simulink model "AdaptiveQ_Function"  (R2025b)
settings: Solver=ode1  StartTime=0.0  StopTime=inf  FixedStep=0.002  RelTol=1e-3  EnableMultiTasking=on
undefined symbols (not defined in the file): A, B, P_ss_vec, Q, R
settings Model: SimulationMode=external  ExtModeTrigDuration=5000  Creator=MLevis  LastModifiedBy=mj
settings SolverCC: AlgebraicLoopSolver=TrustRegion  PositivePriorityOrder=on
settings DataIOCC: LimitDataPoints=on  SaveFormat=Array  SignalLoggingSaveFormat=ModelDataLogs  ReturnWorkspaceOutputs=off
settings OptimizationCC: BooleanDataType=off  OptimizeBlockIOStorage=off  BufferReuse=off  GlobalBufferReuse=off  ExpressionFolding=off  ExpressionDepthLimit=2147483647.0  LocalBlockOutputs=off  InitFltsAndDblsToZero=on  LifeSpan=inf  OptimizeDataStoreBuffers=off  BusAssignmentInplaceUpdate=off
settings DebuggingCC: SaveWithParameterizedLinksMsg=none  UnderspecifiedInitializationDetection=Classic  MergeDetectMultiDrivingBlocksExec=none  SignalResolutionControl=TryResolveAllWithWarning  MultiTaskDSMMsg=warning  MultiTaskCondExecSysMsg=none  FcnCallInpInsideContextMsg=warning  UnconnectedInputMsg=warning  UnconnectedOutputMsg=warning  UnconnectedLineMsg=warning  StateNameClashWarn=warning  SFUnexpectedBacktrackingDiag=warning  SFNoUnconditionalDefaultTransitionDiag=warning  SFExecutionAtInitializationDiag=none  ArithmeticOperatorsInVariantConditions=warning
settings HardwareCC: ProdBitPerPointer=32.0  ProdBitPerSizeT=32.0  ProdBitPerPtrDiffT=32.0  ProdLargestAtomicFloat=None  ProdIntDivRoundTo=Undefined  ProdEndianess=Unspecified  ProdWordSize=32.0  ProdHWDeviceType=32-bit Generic  TargetHWDeviceType=32-bit Generic
settings ModelReferenceCC: EnableRefExpFcnMdlSchedulingChecks=on  PropagateSignalLabelsOutOfModel=off
settings SFSimCC: SimUseLocalCustomCode=off  SimParseCustomCode=off  CustomCodeUndefinedFunction=UseInterfaceOnly
settings RTWCC: SystemTargetFile=quarc_win64.tlc  TemplateMakefile=quarc_default_tmf  RTWUseLocalCustomCode=off  GPUComputeCapability=3.5  DLArmComputeVersion=19.05  Description=QUARC Win64 Target
settings CodeAppCC: StateflowObjectComments=on
settings STFCustomTargetCC: SystemTargetFile=quarc_win64.tlc  TargetPreCompLibLocation=C:\PROGRA~3\QUARC\lib\2020b\win64\release  Debug=off  StopOnOverrun=off
settings GRTTargetCC: ExtMode=on  ExtModeMexFile=quarc_comm  TargetPreCompLibLocation=C:\PROGRA~3\QUARC\lib\2020b\win64\release  TargetLangStandard=C89/C90 (ANSI)  ParMdlRefBuildCompliant=off  CompOptLevelCompliant=off  CombineOutputUpdateFcns=off  MatFileLogging=off  CPPClassGenCompliant=off  GRTInterface=on  UseToolchainInfoCompliant=off
settings ConfigComp: CovMetricSettings=dw  CovSaveCumulativeToWorkspaceVar=on  CovSaveSingleToWorkspaceVar=on  CovExternalEMLEnable=off  CovSFcnEnable=off

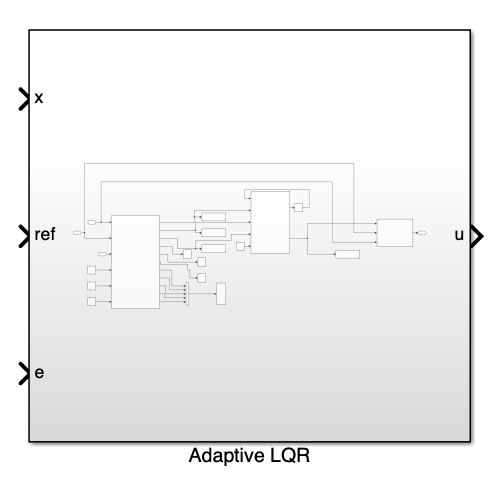
[thumbnail: Simulink's stored preview of the top-level diagram]
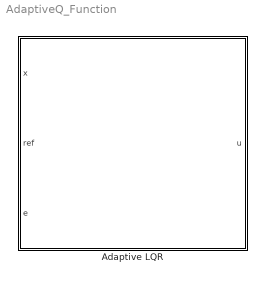
== system AdaptiveQ_Function ==
  Adaptive LQR : Subsystem

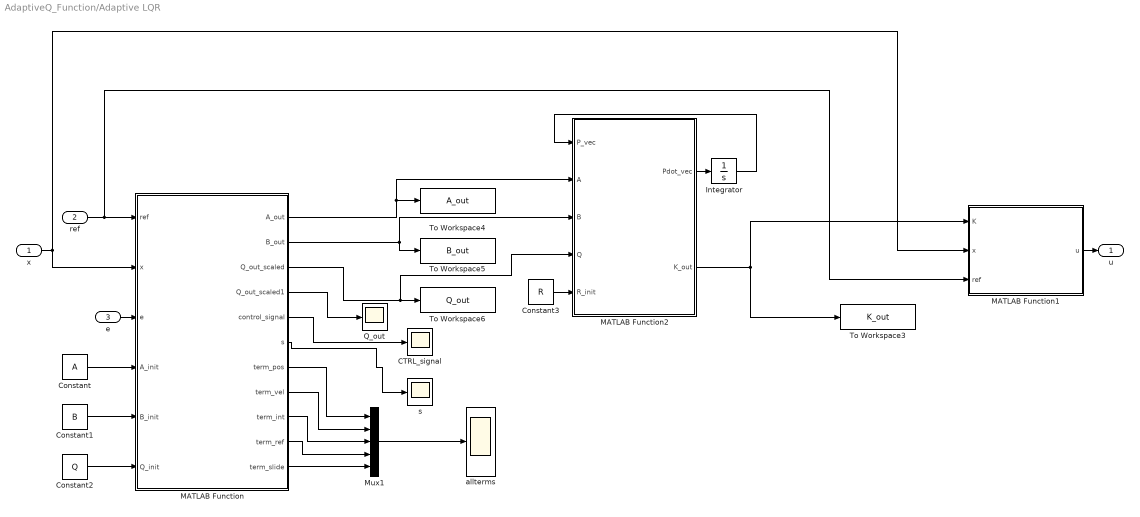
== system AdaptiveQ_Function/Adaptive LQR ==
  x : Inport
  ref : Inport  Port=2
  e : Inport  Port=3
  CTRL_signal : Scope
      settings: ActiveDisplayYMinimum=-1.25  ActiveDisplayYMaximum=1.25  DataLoggingVariableName=ScopeData3
  Constant : Constant  Value=A
  Constant1 : Constant  Value=B
  Constant2 : Constant  Value=Q
  Constant3 : Constant  Value=R
  Integrator : Integrator  InitialCondition=P_ss_vec
  MATLAB Function : MATLAB Function  TreatAsAtomicUnit=on
  MATLAB Function1 : MATLAB Function  TreatAsAtomicUnit=on
  MATLAB Function2 : MATLAB Function  TreatAsAtomicUnit=on
  Mux1 : Mux  Inputs=5
  Q_out : Scope
      settings: ActiveDisplayYMinimum=5.52343  ActiveDisplayYMaximum=110.4974
  To Workspace3 : ToWorkspace  VariableName=K_out  SaveFormat=Structure With Time  SampleTime=-1
  To Workspace4 : ToWorkspace  VariableName=A_out  SaveFormat=Structure With Time  SampleTime=-1
  To Workspace5 : ToWorkspace  VariableName=B_out  SaveFormat=Structure With Time  SampleTime=-1
  To Workspace6 : ToWorkspace  VariableName=Q_out  SaveFormat=Structure With Time  SampleTime=-1
  allterms : Scope
      settings: ActiveDisplayYMinimum=-8.13738  ActiveDisplayYMaximum=73.23642
  s : Scope
      settings: ActiveDisplayYMinimum=-2.95635  ActiveDisplayYMaximum=2.58598  DataLoggingVariableName=ScopeData9
  u : Outport
  wires:
  e/1 -> MATLAB Function/3(e)
  x/1 -> MATLAB Function/2(x), MATLAB Function1/2(x)
  Constant/1 -> MATLAB Function/4(A_init)
  MATLAB Function/3(Q_out_scaled) -> MATLAB Function2/4(Q), To Workspace6/1
  MATLAB Function/2(B_out) -> To Workspace5/1, MATLAB Function2/3(B)
  Mux1/1 -> allterms/1
  MATLAB Function/4(Q_out_scaled1) -> Q_out/1
  MATLAB Function/7(term_pos) -> Mux1/1
  MATLAB Function/1(A_out) -> To Workspace4/1, MATLAB Function2/2(A)
  Constant2/1 -> MATLAB Function/6(Q_init)
  MATLAB Function/8(term_vel) -> Mux1/2
  Constant1/1 -> MATLAB Function/5(B_init)
  MATLAB Function/10(term_ref) -> Mux1/4
  MATLAB Function/11(term_slide) -> Mux1/5
  MATLAB Function/6(s) -> s/1
  MATLAB Function2/2(K_out) -> To Workspace3/1, MATLAB Function1/1(K)
  MATLAB Function1/1(u) -> u/1
  MATLAB Function2/1(Pdot_vec) -> Integrator/1
  MATLAB Function/9(term_int) -> Mux1/3
  MATLAB Function/5(control_signal) -> CTRL_signal/1
  ref/1 -> MATLAB Function1/3(ref), MATLAB Function/1(ref)
  Constant3/1 -> MATLAB Function2/5(R_init)
  Integrator/1 -> MATLAB Function2/1(P_vec)

== matlab function AdaptiveQ_Function/Adaptive LQR/MATLAB Function1 ==
  data: K input; u output; x input; ref input
function u = AdaptiveLQRControl(K, x, ref)
% x = [theta; alpha; theta_dot; alpha_dot]
% ref = desired theta
x_ref = [ref 0 0 0]';
e = x_ref - x;

u = K*e;

%% limit voltage
u = max(min(u, 5), -5);
end

== matlab function AdaptiveQ_Function/Adaptive LQR/MATLAB Function ==
  settings: updateMethod=DISCRETE
  data: ref input; x input; e input; A_init input; B_init input; Q_init input; A_out output; B_out output; Q_out_scaled output; Q_out_scaled1 output; control_signal output; s output; term_pos output; term_vel output; term_int output; term_ref output; term_slide output
function [A_out, B_out, Q_out_scaled, Q_out_scaled1, control_signal, s, ...
          term_pos, term_vel, term_int, term_ref, term_slide] = ...
          AdaptiveQ_QUBE_Simulink(ref, x, e, A_init, B_init, Q_init)
% Adaptive Q for QUBE-2 in Simulink with term logging
%
% Inputs:
%   ref      - reference theta
%   x        - state [theta; alpha; theta_dot; alpha_dot]
%   e        - tracking error (ref - theta)
%   A_init   - initial system A matrix
%   B_init   - initial system B matrix
%   Q_init   - initial Q matrix
%
% Outputs:
%   A_out, B_out          - updated system matrices
%   Q_out_scaled           - updated Q matrix
%   Q_out_scaled1          - scalar Q(1,1)
%   control_signal         - sliding-modulated control signal
%   s                      - sliding variable
%   term_pos, term_vel, term_int, term_ref, term_slide - contributions

%% ---------------- Persistent Variables ----------------
persistent e_int prev_ref x3_filt
if isempty(e_int)
    e_int = 0;                 % soft integral for Q
    prev_ref = ref;
    x3_filt = x(3);
end

%% ---------------- Filter Angular Velocity ----------------
alpha_filt = 0.8;  % smoothing factor
x3_filt = alpha_filt*x3_filt + (1-alpha_filt)*x(3);

%% ---------------- Soft Integral Q ----------------
lambda_int = 0.99;
e_int = lambda_int*e_int + e(1);

%% ---------------- Gains ----------------
k_p = 35;    % position urgency
k_d = 12;    % velocity urgency
k_i = 8;     % integral for bias removal
k_ref = 10;  % reference rate contribution
sliding_scale = 0.5;

%% ---------------- Base Q Contributions ----------------
error_mag = abs(e(1));
term_pos = k_p * error_mag^0.8;
term_pos = min(term_pos, 100);
term_vel = k_d * abs(x3_filt)^0.5;
term_vel = min(term_vel, 100);
term_int = k_i * abs(e_int)^0.5;
term_int = min(term_int, 100);

%% ---------------- Reference Rate Contribution ----------------
ref_dot = ref - prev_ref;
prev_ref = ref;
term_ref = k_ref * abs(ref_dot);
term_ref = min(term_ref, 100);

%% ---------------- Sliding Mode Contribution ----------------
s = e(1) + 0.5*x3_filt;
adpsldlayer = 0.01 + 0.05*abs(e(1));  % adaptive sliding layer
control_signal = tanh(s/adpsldlayer);
term_slide = sliding_scale * abs(control_signal * Q_init(1,1));

%% ---------------- Total Q ----------------
Q11_scaled = Q_init(1,1) + term_pos + term_vel + term_int + term_ref;
Q11_scaled = Q11_scaled * (1 + sliding_scale * abs(control_signal));

%% ---------------- Clamp Q ----------------
Q_out = Q_init;
Q_out(1,1) = min(max(Q_init(1,1), Q11_scaled), 100);

%% ---------------- Output ----------------
Q_out_scaled = Q_out;
Q_out_scaled1 = Q_out(1,1);
A_out = A_init;
B_out = B_init;
end

== matlab function AdaptiveQ_Function/Adaptive LQR/MATLAB Function2 ==
  data: P_vec input; Pdot_vec output; A input; B input; Q input; R_init input; K_out output
function [Pdot_vec, K_out] = Riccati_LQR_Continuous(P_vec, A, B, Q, R_init)
%% Continuous-time Riccati differential equation for adaptive LQR
%
% Inputs:
%   P_vec - current Riccati matrix (vectorized 16x1 for 4x4 system)
%   A,B,Q,R - current system matrices (continuous-time)
%
% Outputs:
%   Pdot_vec - dP/dt in vectorized form
%   K_out    - current continuous-time LQR gain (1x4)

%% Reshape P from vector to matrix
n = size(A,1);
P = reshape(P_vec, n, n);

RC_a = 1; % "RC_a > 1" means Less aggressive controller 
R = R_init * RC_a;

%% ---- Continuous-time Riccati differential equation ----
Pdot = A'*P + P*A - P*B*(R\(B'))*P + Q;

% Optional: accelerate convergence (tune 1–10)
gamma = 1;  
Pdot = gamma * Pdot;

% Optional: numerical clamp to avoid blow-up
Pdot = min(max(Pdot, -1e6), 1e6);

%% ---- Compute continuous-time LQR gain ----
K_mat = (R\(B' * P));

K_max = 100;
K_mat = min(max(K_mat, -K_max), K_max);
%% ---- Outputs ----
Pdot_vec = reshape(Pdot, [], 1);
K_out = K_mat;
end
